simulink model "sf_tetris"  (Simulink 6.0)
settings: Solver=ode5  StartTime=0.0  StopTime=inf  FixedStep=1  RelTol=1e-3
settings Model: CovMetricSettings=dcmtr  Creator=The MathWorks Inc.  LastModifiedBy=batserve  ExtModeAutoUpdateStatusClock=off
settings DataIOCC: SignalLoggingName=sigsOut
settings OptimizationCC: BooleanDataType=off
settings DebuggingCC: CheckExecutionContextPreStartOutputMsg=on  CheckExecutionContextRuntimeOutputMsg=on  SolverPrmCheckMsg=none
settings HardwareCC: TargetUnknown=on

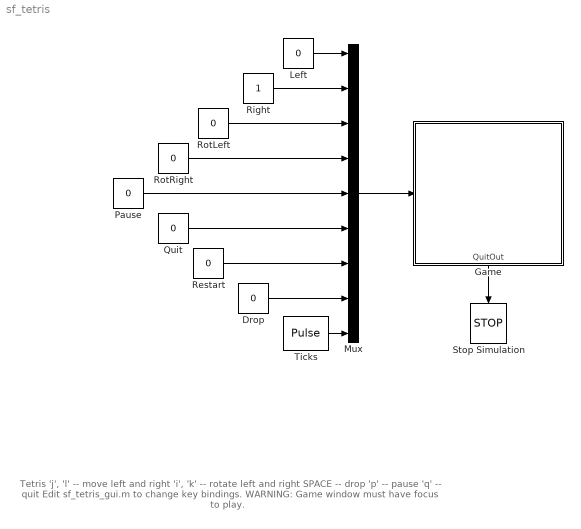
== system sf_tetris ==
  note: Tetris
      |
      | 'j', 'l' -- move   left and right
      | 'i', 'k' -- rotate left and right
      |  SPACE   -- drop
      |
      | 'p'      -- pause
      | 'q'      -- quit
      |
      | Edit sf_tetris_gui.m to change key bindings.
      |
      | WARNING: Game window must have focus to play.
  Drop : Constant  Value=0
  Game : Stateflow chart  Orientation=down  TreatAsAtomicUnit=on  PropExecContextAcrossSSBoundary=on
  Left : Constant  Value=0
      settings: AttributesFormatString=\n\n
  Mux : Mux  Inputs=9
  Pause : Constant  Value=0
  Quit : Constant  Value=0
  Restart : Constant  Value=0
  Right : Constant
  RotLeft : Constant  Value=0
  RotRight : Constant  Value=0
  Stop Simulation : Stop  Orientation=down
  Ticks : DiscretePulseGenerator  PulseType=Time based  PulseWidth=50
  wires:
  Left/1 -> Mux/1
  Right/1 -> Mux/2
  Mux/1 -> Game/Trigger
  RotRight/1 -> Mux/4
  RotLeft/1 -> Mux/3
  Pause/1 -> Mux/5
  Quit/1 -> Mux/6
  Game/1(QuitOut) -> Stop Simulation/1
  Ticks/1 -> Mux/9
  Restart/1 -> Mux/7
  Drop/1 -> Mux/8

== stateflow chart Game ==
  state A
    entry: ml.sf_tetris_gui("paint",level,score);
    exit: t = ml.cputime();
  state c = get(x,y) [function]
    (junction 18) -> (junction 19) : [x>=1 && x<=gridW]
    (junction 19) -> (junction 21) : { c = grid[x][y]; }
    (junction 17) -> (junction 20) : { c = 1; }
    (default) -> (junction 17)
    (junction 17) -> (junction 18) : [y>=1 && y<=gridH]
    (junction 17) -> (junction 56) : [y<1] {c = 0; }
  state e = set(x,y,c) [function]
    (default) -> (junction 12)
    (junction 12) -> (junction 13) : [x>=1 && x<=gridW]
    (junction 13) -> (junction 14) : [y>=1 && y<=gridH]
    (junction 14) -> (junction 15) : { grid[x][y] = c;
        |   ml.sf_tetris_gui("set",y,x,c);
        |  e = 0;
        | }
    (junction 12) -> (junction 16) : { e = 1; }
  state e = show(x,y,s,c) [function]
    (junction 36) -> (junction 39)
    (default) -> (junction 35) : { dx = -1;
        |   dy = -1;
        |   i = 0;
        |   e = 0; }
    (junction 35) -> (junction 36) : [i<16]
    (junction 35) -> (junction 37)
    (junction 36) -> (junction 38) : [(s>>i) & 0x1]
    (junction 43) -> (junction 35)
    (junction 39) -> (junction 40)
    (junction 42) -> (junction 41) : {dx=-1; dy++;}
    (junction 38) -> (junction 39) : { e+=set(x+dx,y+dy,c); }
    (junction 39) -> (junction 42) : [dx==2]
    (junction 40) -> (junction 41) : {dx++;}
    (junction 41) -> (junction 43) : { i++; }
  state r = okay(x,y,s) [function]
    (junction 28) -> (junction 44)
    (junction 27) -> (junction 31)
    (junction 30) -> (junction 28) : { i++; }
    (junction 26) -> (junction 30) : {dx=-1; dy++;}
    (junction 23) -> (junction 30) : {dx++;}
    (junction 24) -> (junction 33) : [r==0]
    (junction 24) -> (junction 31)
    (junction 31) -> (junction 26) : [dx==2]
    (junction 25) -> (junction 24) : { r = (get(x+dx,y+dy)==0); }
    (junction 31) -> (junction 23)
    (junction 27) -> (junction 25) : [(s>>i) & 0x1]
    (junction 44) -> (junction 27) : [i<16]
    (default) -> (junction 44) : { i = 0;
        |   dx = -1;
        |   dy = -1; }
    (junction 44) -> (junction 29)
  state ns = rot(s,right) [function]
    (default) -> (junction 61) : { i = 0;
        |   ns = 0;
        |   ns |= s & 0xffff0000;
        |   y = 0; }
    (junction 61) -> (junction 62) : [y<4]
    (junction 62) -> (junction 63) : { x = 0; }
    (junction 63) -> (junction 64) : [x<4]
    (junction 64) -> (junction 65) : [s>>i & 0x1]
    (junction 70) -> (junction 71) : { nx = (~y) & 0x3;
        |   ny = x; }
    (junction 64) -> (junction 66)
    (junction 66) -> (junction 63) : {x++; i++;}
    (junction 63) -> (junction 61) : {y++;}
    (junction 61) -> (junction 67)
    (junction 65) -> (junction 69) : [right]
    (junction 65) -> (junction 70)
    (junction 68) -> (junction 66)
    (junction 69) -> (junction 71) : { nx = y;
        |   ny = (~x) & 0x3; }
    (junction 71) -> (junction 68) : { ns =ns | (1 << (ny*4 + nx)); }
  state num = clear_rows() [function]
    (default) -> (junction 72) : { y=gridH;
        |   num = 0; }
    (junction 72) -> (junction 73) : [y>=1]
    (junction 77) -> (junction 78) : { num++; }
    (junction 78) -> (junction 72) : { y--; }
    (junction 77) -> (junction 75) : [x<=gridW]
    (junction 75) -> (junction 76) : [get(x,y)]
    (junction 76) -> (junction 77) : { x++; }
    (junction 73) -> (junction 77) : {x=1;}
    (junction 79) -> (junction 78)
    (junction 82) -> (junction 79) : { x=1; }
    (junction 79) -> (junction 80) : [x<=gridW]
    (junction 80) -> (junction 81) : { set(x,y+num,get(x,y)); }
    (junction 81) -> (junction 79) : { x++; }
    (junction 75) -> (junction 74)
    (junction 74) -> (junction 82) : [num!=0]
    (junction 74) -> (junction 78)
    (junction 72) -> (junction 83)
  state P
  state Q
    entry:
    ml.sf_tetris_gui('gameover');
    QuitOut;
  (junction 90) -> A : { ml.sf_tetris_gui("init",gridH,gridW);
      |   x = gridW / 2;
      |   y = -2;
      |   delay = .1;
      |   clearedRows = 0;
      |   tOld = 0;
      |   t= 0;
      |   s = shapes[0];
      |   grid = 0;
      |   level = 0;
      |   score = 0; }
  (junction 88) -> (junction 96) : { offscreen=show(x,y,s,0);
      |   nx = x;
      |   ny = y;
      |   ns = s; }
  (junction 22) -> (junction 46) : Left { nx = x - 1;}
  (junction 22) -> (junction 47) : Right { nx = x + 1;}
  (junction 32) -> A : { show(x,y,s,s>>16); }
  (junction 52) -> (junction 91)
  (junction 89) -> (junction 45) : { ny = y + 1;
      |   tOld = t; }
  (junction 46) -> (junction 48)
  (junction 47) -> (junction 48)
  (junction 48) -> (junction 49) : [okay(nx,ny,ns)]
  (junction 95) -> (junction 50) : {y=ny-1;}
  (junction 49) -> (junction 50) : { x = nx;
      |   s = ns; }
  (junction 45) -> (junction 51) : [okay(nx,ny,s)]
  (junction 51) -> (junction 34) : { y = ny; }
  (junction 53) -> (junction 32)
  (junction 45) -> (junction 52) : { show(x,y,s,s>>16);
      |   score +=5;
      |   clearedRows += clear_rows();
      |   s = shapes[floor(ml.rand() * 6.0)];
      |   y = -2;
      |   x = gridW/2; }
  (junction 55) -> (junction 32)
  (junction 34) -> (junction 53)
  (junction 50) -> (junction 54)
  (junction 54) -> (junction 55)
  (junction 22) -> (junction 57)
  (junction 57) -> (junction 58) : RotLeft { ns = rot(s,1); }
  (junction 57) -> (junction 59) : RotRight {ns = rot(s,0); }
  (junction 58) -> (junction 60)
  (junction 59) -> (junction 60)
  (junction 60) -> (junction 48)
  A -> P : Pause
  P -> A : Pause
  (junction 94) -> (junction 93)
  P -> Q : Quit
  A -> Q : Quit
  A -> (junction 84)
  (junction 84) -> (junction 85) : Ticks
  (junction 84) -> (junction 86)
  (junction 85) -> (junction 87) : [t-tOld >= delay]
  (junction 87) -> (junction 88)
  (junction 85) -> A
  (junction 86) -> (junction 88)
  (junction 96) -> (junction 89) : Ticks
  (default) -> (junction 93) : {shapes[0] = S1;
      |   shapes[1] = S2;
      |   shapes[2] = S3;
      |   shapes[3] = S4;
      |   shapes[4] = S5;
      |   shapes[5] = S6; }
  (junction 91) -> (junction 92) : [clearedRows>10]
  (junction 91) -> (junction 32)
  (junction 92) -> (junction 32) : { clearedRows = 0;
      |   delay *= .75;
      |   level++;}
  A -> (junction 93) : Restart
  (junction 93) -> (junction 90)
  P -> (junction 94) : Restart
  (junction 96) -> (junction 95) : Drop
  (junction 96) -> (junction 22)
  (junction 95) -> (junction 97) : [okay(nx,ny,ns)]
  (junction 97) -> (junction 98) : {ny++;
      |  score++; }
  (junction 98) -> (junction 95)
  (junction 48) -> (junction 50)
  (junction 52) -> Q : [offscreen]
  data: x function_input int32; y function_input int32; c function_output int32; x function_input int32; y function_input int32; c function_input int32; e function_output int32; x function_input int32; y function_input int32; s function_input int32; dx temporary int32; dy temporary int32; i temporary int32; c function_input int32; e function_output int32; x function_input int32; y function_input int32; r function_output boolean =1; i temporary int32; dy temporary int32; dx temporary int32; s function_input int32; s function_input int32; ns function_output int32; x temporary int32; y temporary int32; i temporary int32; nx temporary int32; ny temporary int32; right function_input boolean; num function_output double; x temporary int32; y temporary int32; y local int32 =1; gridW constant int32 =20; gridH constant int32 =60; grid local int8 size=20 60; x local int32 =1; S1 constant int32 =0x202222; nx local int32 =1; ny local int32 =1; shapes local int32 size=6; S2 constant int32 =0x3044c0; S3 constant int32 =0x150360; S4 constant int32 =0x250c60; s local int32; ns local int32; S5 constant int32 =0x3504e0; t local double =1; tOld local double =1; delay local double =1; clearedRows local int32 =1; S6 constant int32 =0x170223; level local int32; score local int32; offscreen local int32 =1
  events: Left input EITHER_EDGE_EVENT; Right input EITHER_EDGE_EVENT; RotLeft input EITHER_EDGE_EVENT; RotRight input EITHER_EDGE_EVENT; Pause input EITHER_EDGE_EVENT; Quit input EITHER_EDGE_EVENT; Restart input EITHER_EDGE_EVENT; Drop input EITHER_EDGE_EVENT; Ticks input EITHER_EDGE_EVENT; QuitOut output EITHER_EDGE_EVENT
